simulink model "cllc_plant"  (R2020b)
settings: Solver=FixedStepDiscrete  StartTime=0.0  StopTime=Inf  FixedStep=stepsize  RelTol=1e-3  EnableMultiTasking=on
values from neighbouring files (symbols this model uses):
  Lm1 = Ln*LrP1    (= 0.00016)    [CLLC_Plant_Parameters.m]
  n = 20.0/9.0    (= 2.22222222222)    [CLLC_Plant_Parameters.m]
  stepsize = 2.0E-7    [cllc_data_lib.sldd]
  var_dir_v2g = 0.0    [cllc_data_lib.sldd]
  var_ref_iout = 18.5    [cllc_data_lib.sldd]
  var_ref_vout = 250.0    [cllc_data_lib.sldd]
libraries: fl_lib x219, ee_lib x151, nesl_utility x117, powerlib_meascontrol x15, eeStairGenerator x1
(part 7 of 8)

== system cllc_plant/cllc2/QDsec ==
  VGS : Inport
  Controlled Voltage Source : fl_lib/Electrical/Electrical Sources/Controlled Voltage Source
  Diode3 : ee_lib/Semiconductors & Converters/Diode  Commented=on  ModelType=ee.enum.diode.modelType.pwl  IfMat=[.07, .12, .19, 1.75, 4.24, 7.32, 11.2; .16, .3, .72, 2.14, 4.02, 6.35, 9.12] A  TjVec=[25, 125] degC  VfVec=[.5, .7, .9, 1.3, 1.7, 2.1, 2.5] V  Vf=0.6 V  Ron=0.3 Ohm  Goff=1e-8 S  prmExp=ee.enum.diode.expParam.useTwo  I12=[.0137, .545] A  V12=[.6, .7] V  IS=1e-12 A  ec=1  I1=0.0137 A  V1=0.6 V  RS=0 Ohm  Tmeas=25 degC  N_series=1  N_parallel=1  Rz=0.3 Ohm  BV=inf V  C_param=ee.enum.diode.capParam.fixed  CJ=5 pF  CJ0=5 pF  VJ=1 V  Mgrad=0.5  Vvec=[.1, 10, 100] V  Cvec=[3.5, 1, .4] pF  FC=0.5  Q_param=ee.enum.diode.recoveryParam.off  iRM=-7.15 A  iF=4 A  didt=-750 A/us  trr_factor=3  trr=115 ns  Qrr=1500 s*uA  TT=50 ns  tau=100 ns  T_param=ee.enum.diode.temperatureParam.off  IS_T2=1.25e-7 A  I1_T2=0.245 A  V1_T2=0.5 V  Tmeas2=125 degC  EG_param=ee.enum.diode.egapParam.material_si  EG=1.11 eV  XTI_param=ee.enum.diode.xtiParam.pn  XTI=3  dBVdT=0 V/K  Tdevice=25 degC  i_specify=off  i_priority=None  i=0 A  i_nominal_specify=off  i_nominal_unit=A  i_nominal_value=1  v_specify=off  v_priority=None  v=0 V  v_nominal_specify=off  v_nominal_unit=V  v_nominal_value=1  i_capacitor_specify=off  i_capacitor_priority=None  i_capacitor=0 A  i_capacitor_nominal_specify=off  i_capacitor_nominal_unit=A  i_capacitor_nominal_value=1  v_capacitor_specify=off  v_capacitor_priority=None  v_capacitor=0 V  v_capacitor_nominal_specify=off  v_capacitor_nominal_unit=V  v_capacitor_nominal_value=1  power_dissipated_specify=off  power_dissipated_priority=None  power_dissipated=0 W  power_dissipated_nominal_specify=off  power_dissipated_nominal_unit=W  power_dissipated_nominal_value=1  thermal_network_parameterization=ee.enum.thermalNetworkTopology.cauer  Rth=[0, 10] K/W  Rth_Foster=[4, 6] K/W  thermal_mass_parameterization=ee.enum.thermalNetwork.timeconstant  thermal_mass=[0, 1] J/K  thermal_mass_Foster=[1.5, 3] J/K  thermal_time_constant=[0, 10] s  thermal_time_constant_Foster=[6, 18] s  thermal_mass_initial_temperatures=[25, 25] degC
  F4-23MR12W1M1_B9 : ee_lib/Semiconductors & Converters/N-Channel MOSFET  paramTerminal=ee.enum.mosfet.numberOfTerminals.three  parameterization=1  prmDatasheet=2  prmEquCoeff=1  Beta=5.0 A/V^2  Rds=0.0225 Ohm  Id=50 A  Vgs=15 V  Vth=4.5 V  Vth0=1.7 V  lam=0 1/V  gamma_vth=0.5 V^0.50000  phib=0.5 V  Vth1=1.9071 V  Vbs1=-1 V  Vth2=2.066 V  Vbs2=-2 V  Tmeas=25 degC  RS=0.0001 Ohm  RD=0.0001 Ohm  RB=0.001 Ohm  C_param=1  C_GS=270 pF  C_GD=80 pF  C_DS=0 pF  C_iss=3.68 nF  C_rss=0.028 nF  C_oss=0.22 nF  charge_linearity_param=2  C_OX=200 pF  V_C_OX=-0.5 V  C_iss_vec=[2200,2000,1950,1900,1900,1900,1900,1900,1900,1900,1900,1900,1900,1900,1900,1900,1900,1900,1900,1900,1900] pF  C_rss_vec=[400,200,65,50,43,38,35,33,31,29,28,27,21,18,16,15,14,14,14,14,14] pF  C_oss_vec=[1900,1200,700,550,450,400,350,340,310,290,280,260,200,160,140,120,120,115,110,110,110] pF  C_GS_vec=[270, 300, 290, 280, 295, 255] pF  C_GD_vec=[450, 400, 300, 190, 95, 55] pF  C_DS_vec=[450, 410, 390, 230, 175, 115] pF  C_Vds_vec=[1,5,10,20,30,40,50,60,70,80,90,100,200,300,400,500,600,700,800,900,1000] V  V_GS_for_cap_data=0 V  charge_linearity_param_vgb=ee.enum.mosfet.cgbLinearity.instantly  IsDiode=0 A  Vbi=4.6 V  n=1  Cj0Diode=0 nF  TT=50e-9 s  dVth_dT=-6 mV/K  dVth0_dT=-6 mV/K  Rds_T2=0.033 Ohm  Tmeas2=150 degC  BEXDatasheet=-1.5  BEXEquCoeff=-1.5  etaisDatasheet=3  etaisEquCoeff=3  TdeviceDatasheet=25 degC  TdeviceEquCoeff=25 degC  thermal_network_parameterization=ee.enum.thermalNetworkTopology.cauer  Rth=[0.51, 10] K/W  Rth_Foster=[4, 6] K/W  thermal_mass_parameterization=ee.enum.thermalNetwork.timeconstant  thermal_mass=[0, 1] J/K  thermal_mass_Foster=[1.5, 3] J/K  thermal_time_constant=[0, 10] s  thermal_time_constant_Foster=[6, 18] s  thermal_mass_initial_temperatures=[25, 25] degC  betaref=18 A/V^2  Vfbref=-1.1 V  gamma=3.5 V^0.50000  phib2ref=1 V  thesatref=0.4 1/V  alpha=0  Vp=5e-2 V  thesrref=0 1/V  m=8  Tref=25 degC  Cox=1500 pF  Cgso=100 pF  Cgdo=14 pF  Rsref=2e-3 Ohm  Rdref=0.17 Ohm  Rgref=8.4 Ohm  Rbref=2e-3 Ohm  Isref=5.2e-13 A  Cj0=480 pF  Tprm=1  etabet=1.3  Stvfb=5e-4 V/K  Stphib=-8.5e-4 V/K  etasat=1.04  etasr=0.65  etar=0.95  etais=3  Tsim=25 degC  T0=[25, 25] degC
      settings: LogSimulationData=on
  ILm9 : fl_lib/Electrical/Electrical Sensors/Current Sensor
  PS-Simulink Converter22 : nesl_utility/PS-Simulink Converter  PhysicalDomain=network_engine_domain  SubClassName=ps_output  LeftPortType=input  RightPortType=output  PseudoPeriodic=off  Frequencies=[]  Unit=1  AffineConversion=off
  PS-Simulink Converter25 : nesl_utility/PS-Simulink Converter  PhysicalDomain=network_engine_domain  SubClassName=ps_output  LeftPortType=input  RightPortType=output  PseudoPeriodic=off  Frequencies=[]  Unit=1  AffineConversion=off
  Rg : ee_lib/Passive/Resistor  R=2 Ohm  R_tol=1  enable_R_tol=0  tol_distribution=1  nSigma=4  enable_operating_limits=0  operating_limit_action=2  max_working_voltage=100 V  power_rating=1 W  enable_faults=0  fault_action=1  R_faulted=inf Ohm  enable_temporal_fault=0  t_fault=1 s  enable_behavioral_fault=0  max_permissible_current=1 A  t_fail_on_current=1 s  noise_mode=0  sample_time=1e-3 s  repeatability=1  auto_seed=2919300768  user_seed=0  Tdevice=25 degC  alpha=3.93e-3 1/K  Tmeas=25 degC  thermal_mass=100 J/K  power_derating_T1=70 degC  power_derating_T2=155 degC  operating_temperature_range_vec=[-50, 150] degC  temperature_specify=off  temperature_priority=High  temperature=298.15 K  temperature_nominal_specify=off  temperature_nominal_unit=K  temperature_nominal_value=1
  Simulink-PS Converter2 : nesl_utility/Simulink-PS Converter  PhysicalDomain=network_engine_domain  SubClassName=ps_input  LeftPortType=input  RightPortType=output  PseudoPeriodic=off  Frequencies=[]  NoiseDistribution=none  NoiseParameters=[]  Unit=1  AffineConversion=off  FilteringAndDerivatives=provide  SimscapeFilterOrder=1  InputFilterTimeConstant=0.001  UdotUserProvided=0
  Voltage Sensor17 : fl_lib/Electrical/Electrical Sensors/Voltage Sensor
  + : PMIOPort  Side=Left
  - : PMIOPort  Port=2  Side=Left
  VDS : Outport  VectorParamsAs1DForOutWhenUnconnected=off
  IDS : Outport  Port=2  VectorParamsAs1DForOutWhenUnconnected=off
  wires:
  PS-Simulink Converter22/1 -> IDS/1
  PS-Simulink Converter25/1 -> VDS/1
  VGS/1 -> Simulink-PS Converter2/1
  connections:
  F4-23MR12W1M1_B9/LConn1 -- Rg/RConn1
  F4-23MR12W1M1_B9/RConn1 -- ILm9/RConn2 -- Voltage Sensor17/LConn1 -- Diode3/RConn1
  +/RConn1 -- ILm9/LConn1
  Controlled Voltage Source/RConn2 -- F4-23MR12W1M1_B9/RConn2 -- Voltage Sensor17/RConn2 -- Diode3/LConn1 -- -/RConn1
  PS-Simulink Converter22/LConn1 -- ILm9/RConn1
  PS-Simulink Converter25/LConn1 -- Voltage Sensor17/RConn1
  Rg/LConn1 -- Controlled Voltage Source/LConn1
  Controlled Voltage Source/RConn1 -- Simulink-PS Converter2/RConn1

== system cllc_plant/cllc2/tank_current_pri ==
  note: 1) Add Subsystem or Model blocks as valid variant choices.
      | 2) You cannot connect blocks at this level. At simulation, connectivity is automatically
      | determined, based on the active variant and port name matching.
  G2V : Subsystem  VariantControl=var_dir_v2g==0
  V2G : Subsystem  VariantControl=var_dir_v2g==1
  L : PMIOPort  Side=Left
  R : PMIOPort  Port=2  Side=Left
  to_scope : Outport

== system cllc_plant/cllc2/tank_current_sec ==
  note: 1) Add Subsystem or Model blocks as valid variant choices.
      | 2) You cannot connect blocks at this level. At simulation, connectivity is automatically
      | determined, based on the active variant and port name matching.
  G2V : Subsystem  VariantControl=var_dir_v2g==0
  V2G : Subsystem  VariantControl=var_dir_v2g==1
  L : PMIOPort  Side=Left
  R : PMIOPort  Port=2  Side=Left
  to_scope : Outport

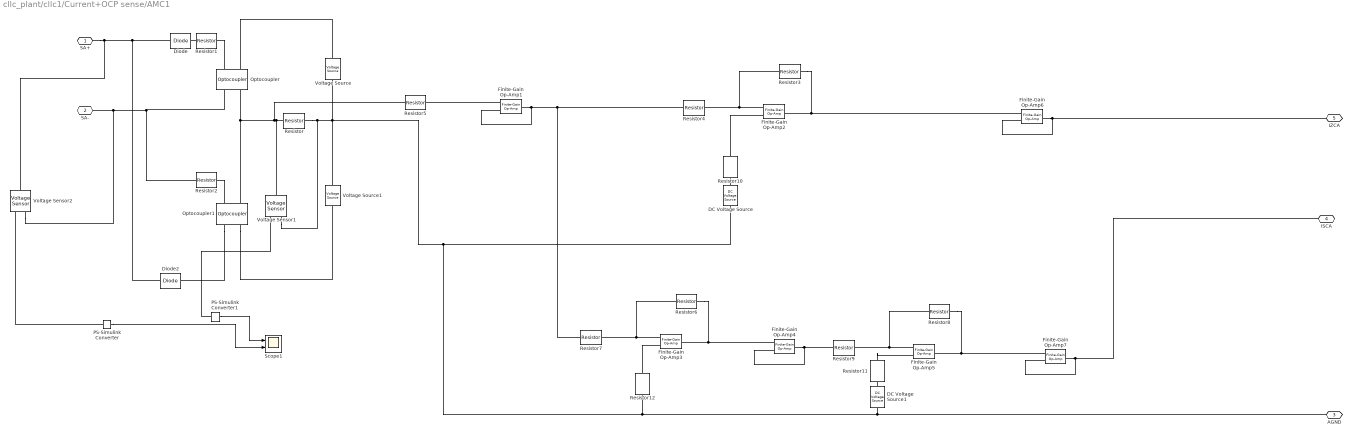
== system cllc_plant/cllc1/Current+OCP sense/AMC1 ==
  DC Voltage Source : fl_lib/Electrical/Electrical Sources/DC Voltage Source  v0=0.745 V
  DC Voltage Source1 : fl_lib/Electrical/Electrical Sources/DC Voltage Source  v0=0.745 V
  Diode : fl_lib/Electrical/Electrical Elements/Diode  Vf=0.000001 V  Ron=0.0000001 Ohm  Goff=1e-8 1/Ohm  i_specify=off  i_priority=None  i=0 A  i_nominal_specify=off  i_nominal_unit=A  i_nominal_value=1  v_specify=off  v_priority=None  v=0 V  v_nominal_specify=off  v_nominal_unit=V  v_nominal_value=1
  Diode2 : fl_lib/Electrical/Electrical Elements/Diode  Vf=0.000001 V  Ron=0.0000001 Ohm  Goff=1e-8 1/Ohm  i_specify=off  i_priority=None  i=0 A  i_nominal_specify=off  i_nominal_unit=A  i_nominal_value=1  v_specify=off  v_priority=None  v=0 V  v_nominal_specify=off  v_nominal_unit=V  v_nominal_value=1
  Finite-Gain Op-Amp1 : ee_lib/Integrated Circuits/Finite-Gain Op-Amp  A=1000  Rin=1e6 Ohm  Rout=100 Ohm  Vmin=-3.65 V  Vmax=3.65 V  noise_mode=0  v_noise=30e-9 V/Hz^0.50000  noise_prm=1  i_noise=0.5e-12 A/Hz^0.50000  ip_noise=0.5e-12 A/Hz^0.50000  in_noise=0.5e-12 A/Hz^0.50000  sample_time=1e-3 s  repeatability=1  auto_seed_v=3726858180  auto_seed_ip=508128604  auto_seed_in=167602409  user_seed_v=0  user_seed_ip=0  user_seed_in=0
      settings: SourceProductBaseCode=PS  InternalSimscapePortConfiguration="{\"Bottom\":[],\"Left\":[{\"id\":\"p\",\"label\":\"+\",\"type\":\"foundation.electrical.electrical\"},{\"id\":\"n\",\"label\":\"-\",\"type\":\"foundation.electrical.electrical\"}],\"Right\":[{\"id\":\"out\",\"label\":\"\",\"type\":\"foundation.electrical.electrical\"}],\"Top\":[]}"
  Finite-Gain Op-Amp2 : ee_lib/Integrated Circuits/Finite-Gain Op-Amp  A=1000  Rin=1e6 Ohm  Rout=100 Ohm  Vmin=0 V  Vmax=3.65 V  noise_mode=0  v_noise=30e-9 V/Hz^0.50000  noise_prm=1  i_noise=0.5e-12 A/Hz^0.50000  ip_noise=0.5e-12 A/Hz^0.50000  in_noise=0.5e-12 A/Hz^0.50000  sample_time=1e-3 s  repeatability=1  auto_seed_v=2569225923  auto_seed_ip=2595506743  auto_seed_in=2218060313  user_seed_v=0  user_seed_ip=0  user_seed_in=0
      settings: SourceProductBaseCode=PS  InternalSimscapePortConfiguration="{\"Bottom\":[],\"Left\":[{\"id\":\"p\",\"label\":\"+\",\"type\":\"foundation.electrical.electrical\"},{\"id\":\"n\",\"label\":\"-\",\"type\":\"foundation.electrical.electrical\"}],\"Right\":[{\"id\":\"out\",\"label\":\"\",\"type\":\"foundation.electrical.electrical\"}],\"Top\":[]}"
  Finite-Gain Op-Amp3 : ee_lib/Integrated Circuits/Finite-Gain Op-Amp  A=1000  Rin=1e6 Ohm  Rout=100 Ohm  Vmin=-3.65 V  Vmax=3.65 V  noise_mode=0  v_noise=30e-9 V/Hz^0.50000  noise_prm=1  i_noise=0.5e-12 A/Hz^0.50000  ip_noise=0.5e-12 A/Hz^0.50000  in_noise=0.5e-12 A/Hz^0.50000  sample_time=1e-3 s  repeatability=1  auto_seed_v=32244056  auto_seed_ip=2958946266  auto_seed_in=4063126573  user_seed_v=0  user_seed_ip=0  user_seed_in=0
      settings: SourceProductBaseCode=PS  InternalSimscapePortConfiguration="{\"Bottom\":[],\"Left\":[{\"id\":\"p\",\"label\":\"+\",\"type\":\"foundation.electrical.electrical\"},{\"id\":\"n\",\"label\":\"-\",\"type\":\"foundation.electrical.electrical\"}],\"Right\":[{\"id\":\"out\",\"label\":\"\",\"type\":\"foundation.electrical.electrical\"}],\"Top\":[]}"
  Finite-Gain Op-Amp4 : ee_lib/Integrated Circuits/Finite-Gain Op-Amp  A=1000  Rin=1e6 Ohm  Rout=100 Ohm  Vmin=-3.65 V  Vmax=3.65 V  noise_mode=0  v_noise=30e-9 V/Hz^0.50000  noise_prm=1  i_noise=0.5e-12 A/Hz^0.50000  ip_noise=0.5e-12 A/Hz^0.50000  in_noise=0.5e-12 A/Hz^0.50000  sample_time=1e-3 s  repeatability=1  auto_seed_v=3751810512  auto_seed_ip=486518659  auto_seed_in=1522863725  user_seed_v=0  user_seed_ip=0  user_seed_in=0
      settings: SourceProductBaseCode=PS  InternalSimscapePortConfiguration="{\"Bottom\":[],\"Left\":[{\"id\":\"p\",\"label\":\"+\",\"type\":\"foundation.electrical.electrical\"},{\"id\":\"n\",\"label\":\"-\",\"type\":\"foundation.electrical.electrical\"}],\"Right\":[{\"id\":\"out\",\"label\":\"\",\"type\":\"foundation.electrical.electrical\"}],\"Top\":[]}"
  Finite-Gain Op-Amp5 : ee_lib/Integrated Circuits/Finite-Gain Op-Amp  A=1000  Rin=1e6 Ohm  Rout=100 Ohm  Vmin=0 V  Vmax=3.65 V  noise_mode=0  v_noise=30e-9 V/Hz^0.50000  noise_prm=1  i_noise=0.5e-12 A/Hz^0.50000  ip_noise=0.5e-12 A/Hz^0.50000  in_noise=0.5e-12 A/Hz^0.50000  sample_time=1e-3 s  repeatability=1  auto_seed_v=1039110775  auto_seed_ip=2406613241  auto_seed_in=2631642888  user_seed_v=0  user_seed_ip=0  user_seed_in=0
      settings: SourceProductBaseCode=PS  InternalSimscapePortConfiguration="{\"Bottom\":[],\"Left\":[{\"id\":\"p\",\"label\":\"+\",\"type\":\"foundation.electrical.electrical\"},{\"id\":\"n\",\"label\":\"-\",\"type\":\"foundation.electrical.electrical\"}],\"Right\":[{\"id\":\"out\",\"label\":\"\",\"type\":\"foundation.electrical.electrical\"}],\"Top\":[]}"
  Finite-Gain Op-Amp6 : ee_lib/Integrated Circuits/Finite-Gain Op-Amp  A=1000  Rin=1e6 Ohm  Rout=100 Ohm  Vmin=-3.65 V  Vmax=3.65 V  noise_mode=0  v_noise=30e-9 V/Hz^0.50000  noise_prm=1  i_noise=0.5e-12 A/Hz^0.50000  ip_noise=0.5e-12 A/Hz^0.50000  in_noise=0.5e-12 A/Hz^0.50000  sample_time=1e-3 s  repeatability=1  auto_seed_v=1291965207  auto_seed_ip=3427992560  auto_seed_in=3417254766  user_seed_v=0  user_seed_ip=0  user_seed_in=0
      settings: SourceProductBaseCode=PS  InternalSimscapePortConfiguration="{\"Bottom\":[],\"Left\":[{\"id\":\"p\",\"label\":\"+\",\"type\":\"foundation.electrical.electrical\"},{\"id\":\"n\",\"label\":\"-\",\"type\":\"foundation.electrical.electrical\"}],\"Right\":[{\"id\":\"out\",\"label\":\"\",\"type\":\"foundation.electrical.electrical\"}],\"Top\":[]}"
  Finite-Gain Op-Amp7 : ee_lib/Integrated Circuits/Finite-Gain Op-Amp  A=1000  Rin=1e6 Ohm  Rout=100 Ohm  Vmin=-3.65 V  Vmax=3.65 V  noise_mode=0  v_noise=30e-9 V/Hz^0.50000  noise_prm=1  i_noise=0.5e-12 A/Hz^0.50000  ip_noise=0.5e-12 A/Hz^0.50000  in_noise=0.5e-12 A/Hz^0.50000  sample_time=1e-3 s  repeatability=1  auto_seed_v=3354765737  auto_seed_ip=1507956285  auto_seed_in=233205360  user_seed_v=0  user_seed_ip=0  user_seed_in=0
      settings: SourceProductBaseCode=PS  InternalSimscapePortConfiguration="{\"Bottom\":[],\"Left\":[{\"id\":\"p\",\"label\":\"+\",\"type\":\"foundation.electrical.electrical\"},{\"id\":\"n\",\"label\":\"-\",\"type\":\"foundation.electrical.electrical\"}],\"Right\":[{\"id\":\"out\",\"label\":\"\",\"type\":\"foundation.electrical.electrical\"}],\"Top\":[]}"
  Optocoupler : ee_lib/Semiconductors & Converters/Optocoupler  CTR=8.2  prmExp=1  I12=[.001, .002] A  V12=[0.000001, 0.000002] V  IS=1e-10 A  ec=2  RS=0.000001 Ohm  Tmeas=25 degC  C_param=1  CJ=0.000001 pF  CJ0=5 pF  VJ=1 V  Mgrad=0.5  Vvec=[.1, 10, 100] V  Cvec=[3.5, 1, .4] pF  FC=0.5  T_param=1  IS_T2=1.8e-8 A  I1_T2=0.029 A  V1_T2=1.05 V  Tmeas2=125 degC  EG_param=1  EG=1.11 eV  XTI_param=1  XTI=3  Tdevice=25 degC  i_capacitor_specify=off  i_capacitor_priority=High  i_capacitor=0 A  i_capacitor_nominal_specify=off  i_capacitor_nominal_unit=A  i_capacitor_nominal_value=1  v_capacitor_specify=off  v_capacitor_priority=None  v_capacitor=0 V  v_capacitor_nominal_specify=off  v_capacitor_nominal_unit=V  v_capacitor_nominal_value=1  thermal_network_parameterization=ee.enum.thermalNetworkTopology.cauer  Rth=[0, 10] K/W  Rth_Foster=[4, 6] K/W  thermal_mass_parameterization=ee.enum.thermalNetwork.timeconstant  thermal_mass=[0, 1] J/K  thermal_mass_Foster=[1.5, 3] J/K  thermal_time_constant=[0, 10] s  thermal_time_constant_Foster=[6, 18] s  thermal_mass_initial_temperatures=[25, 25] degC
      settings: SourceProductBaseCode=PS  InternalSimscapePortConfiguration="{\"Bottom\":[],\"Left\":[{\"id\":\"p\",\"label\":\"\",\"type\":\"foundation.electrical.electrical\"},{\"id\":\"C\",\"label\":\"\",\"type\":\"foundation.electrical.electrical\"}],\"Right\":[{\"id\":\"n\",\"label\":\"\",\"type\":\"foundation.electrical.electrical\"},{\"id\":\"E\",\"label\":\"\",\"type\":\"foundation.electrical.electrical\"}],\"Top\":[]}"
  Optocoupler1 : ee_lib/Semiconductors & Converters/Optocoupler  CTR=8.2  prmExp=1  I12=[.001, .002] A  V12=[0.000001, 0.000002] V  IS=1e-10 A  ec=2  RS=0.000001 Ohm  Tmeas=25 degC  C_param=1  CJ=0.000001 pF  CJ0=5 pF  VJ=1 V  Mgrad=0.5  Vvec=[.1, 10, 100] V  Cvec=[3.5, 1, .4] pF  FC=0.5  T_param=1  IS_T2=1.8e-8 A  I1_T2=0.029 A  V1_T2=1.05 V  Tmeas2=125 degC  EG_param=1  EG=1.11 eV  XTI_param=1  XTI=3  Tdevice=25 degC  i_capacitor_specify=off  i_capacitor_priority=High  i_capacitor=0 A  i_capacitor_nominal_specify=off  i_capacitor_nominal_unit=A  i_capacitor_nominal_value=1  v_capacitor_specify=off  v_capacitor_priority=None  v_capacitor=0 V  v_capacitor_nominal_specify=off  v_capacitor_nominal_unit=V  v_capacitor_nominal_value=1  thermal_network_parameterization=ee.enum.thermalNetworkTopology.cauer  Rth=[0, 10] K/W  Rth_Foster=[4, 6] K/W  thermal_mass_parameterization=ee.enum.thermalNetwork.timeconstant  thermal_mass=[0, 1] J/K  thermal_mass_Foster=[1.5, 3] J/K  thermal_time_constant=[0, 10] s  thermal_time_constant_Foster=[6, 18] s  thermal_mass_initial_temperatures=[25, 25] degC
      settings: SourceProductBaseCode=PS  InternalSimscapePortConfiguration="{\"Bottom\":[],\"Left\":[{\"id\":\"p\",\"label\":\"\",\"type\":\"foundation.electrical.electrical\"},{\"id\":\"C\",\"label\":\"\",\"type\":\"foundation.electrical.electrical\"}],\"Right\":[{\"id\":\"n\",\"label\":\"\",\"type\":\"foundation.electrical.electrical\"},{\"id\":\"E\",\"label\":\"\",\"type\":\"foundation.electrical.electrical\"}],\"Top\":[]}"
  PS-Simulink Converter : nesl_utility/PS-Simulink Converter  PhysicalDomain=network_engine_domain  SubClassName=ps_output  LeftPortType=input  RightPortType=output  PseudoPeriodic=off  Frequencies=[]  Unit=1  AffineConversion=off
  PS-Simulink Converter1 : nesl_utility/PS-Simulink Converter  PhysicalDomain=network_engine_domain  SubClassName=ps_output  LeftPortType=input  RightPortType=output  PseudoPeriodic=off  Frequencies=[]  Unit=1  AffineConversion=off
  Resistor : fl_lib/Electrical/Electrical Elements/Resistor  R=50 Ohm  i_specify=off  i_priority=None  i=0 A  i_nominal_specify=off  i_nominal_unit=A  i_nominal_value=1  v_specify=off  v_priority=None  v=0 V  v_nominal_specify=off  v_nominal_unit=V  v_nominal_value=1
  Resistor1 : fl_lib/Electrical/Electrical Elements/Resistor  R=100 Ohm  i_specify=off  i_priority=None  i=0 A  i_nominal_specify=off  i_nominal_unit=A  i_nominal_value=1  v_specify=off  v_priority=None  v=0 V  v_nominal_specify=off  v_nominal_unit=V  v_nominal_value=1
  Resistor{3..12} (10 alike) : fl_lib/Electrical/Electrical Elements/Resistor  R=1000 Ohm  i_specify=off  i_priority=None  i=0 A  i_nominal_specify=off  i_nominal_unit=A  i_nominal_value=1  v_specify=off  v_priority=None  v=0 V  v_nominal_specify=off  v_nominal_unit=V  v_nominal_value=1
  Resistor2 : fl_lib/Electrical/Electrical Elements/Resistor  R=100 Ohm  i_specify=off  i_priority=None  i=0 A  i_nominal_specify=off  i_nominal_unit=A  i_nominal_value=1  v_specify=off  v_priority=None  v=0 V  v_nominal_specify=off  v_nominal_unit=V  v_nominal_value=1
  Scope1 : Scope  NumInputPorts=2
  Voltage Sensor1 : fl_lib/Electrical/Electrical Sensors/Voltage Sensor
  Voltage Sensor2 : fl_lib/Electrical/Electrical Sensors/Voltage Sensor
  Voltage Source : ee_lib/Sources/Voltage Source  dc_voltage=3.6 V  ac_voltage=0 V  ac_shift=0 rad  ac_frequency=60 Hz  noise_mode=0  PSD=0 V^2/Hz  repeatability=1  auto_seed=3043863152  user_seed=0  sample_time=1e-3 s  i_specify=off  i_priority=None  i=0 A  i_nominal_specify=off  i_nominal_unit=A  i_nominal_value=1  v_specify=off  v_priority=None  v=0 V  v_nominal_specify=off  v_nominal_unit=V  v_nominal_value=1
  Voltage Source1 : ee_lib/Sources/Voltage Source  dc_voltage=3.6 V  ac_voltage=0 V  ac_shift=0 rad  ac_frequency=60 Hz  noise_mode=0  PSD=0 V^2/Hz  repeatability=1  auto_seed=4264595182  user_seed=0  sample_time=1e-3 s  i_specify=off  i_priority=None  i=0 A  i_nominal_specify=off  i_nominal_unit=A  i_nominal_value=1  v_specify=off  v_priority=None  v=0 V  v_nominal_specify=off  v_nominal_unit=V  v_nominal_value=1
  SA+ : PMIOPort  Side=Left
  SA- : PMIOPort  Port=2  Side=Left
  AGND : PMIOPort  Port=3  Side=Left
  ISCA : PMIOPort  Port=4  Side=Right
  IZCA : PMIOPort  Port=5  Side=Right
  wires:
  PS-Simulink Converter1/1 -> Scope1/1
  PS-Simulink Converter/1 -> Scope1/2
  connections:
  Resistor7/RConn1 -- Resistor6/LConn1 -- Finite-Gain Op-Amp3/LConn2
  Resistor2/RConn1 -- Optocoupler1/LConn1
  Diode2/RConn1 -- Diode/LConn1 -- SA+/RConn1 -- Voltage Sensor2/LConn1
  Resistor6/RConn1 -- Finite-Gain Op-Amp4/LConn1 -- Finite-Gain Op-Amp3/RConn1
  Finite-Gain Op-Amp1/RConn1 -- Resistor4/LConn1 -- Resistor7/LConn1 -- Finite-Gain Op-Amp1/LConn2
  ISCA/RConn1 -- Finite-Gain Op-Amp7/RConn1 -- Finite-Gain Op-Amp7/LConn2
  SA-/RConn1 -- Resistor2/LConn1 -- Optocoupler/RConn1 -- Voltage Sensor2/RConn2
  Resistor1/LConn1 -- Diode/RConn1
  Finite-Gain Op-Amp2/LConn2 -- Resistor4/RConn1 -- Resistor3/LConn1
  Optocoupler1/RConn1 -- Diode2/LConn1
  Resistor1/RConn1 -- Optocoupler/LConn1
  IZCA/RConn1 -- Finite-Gain Op-Amp6/LConn2 -- Finite-Gain Op-Amp6/RConn1
  Optocoupler1/RConn2 -- Voltage Source1/RConn1
  Resistor10/LConn1 -- Finite-Gain Op-Amp2/LConn1
  Finite-Gain Op-Amp4/LConn2 -- Resistor9/LConn1 -- Finite-Gain Op-Amp4/RConn1
  Optocoupler1/LConn2 -- Optocoupler/RConn2 -- Resistor5/LConn1 -- Resistor/LConn1 -- Voltage Sensor1/LConn1
  Voltage Source/LConn1 -- Optocoupler/LConn2
  Resistor3/RConn1 -- Finite-Gain Op-Amp6/LConn1 -- Finite-Gain Op-Amp2/RConn1
  Resistor9/RConn1 -- Resistor8/LConn1 -- Finite-Gain Op-Amp5/LConn2
  Finite-Gain Op-Amp1/LConn1 -- Resistor5/RConn1
  Resistor8/RConn1 -- Finite-Gain Op-Amp7/LConn1 -- Finite-Gain Op-Amp5/RConn1
  Resistor12/LConn1 -- Finite-Gain Op-Amp3/LConn1
  PS-Simulink Converter/LConn1 -- Voltage Sensor2/RConn1
  PS-Simulink Converter1/LConn1 -- Voltage Sensor1/RConn1
  DC Voltage Source/LConn1 -- Resistor10/RConn1
  Resistor11/RConn1 -- DC Voltage Source1/LConn1
  Resistor11/LConn1 -- Finite-Gain Op-Amp5/LConn1
  DC Voltage Source/RConn1 -- AGND/RConn1 -- DC Voltage Source1/RConn1 -- Resistor12/RConn1 -- Voltage Source/RConn1 -- Voltage Source1/LConn1 -- Resistor/RConn1 -- Voltage Sensor1/RConn2

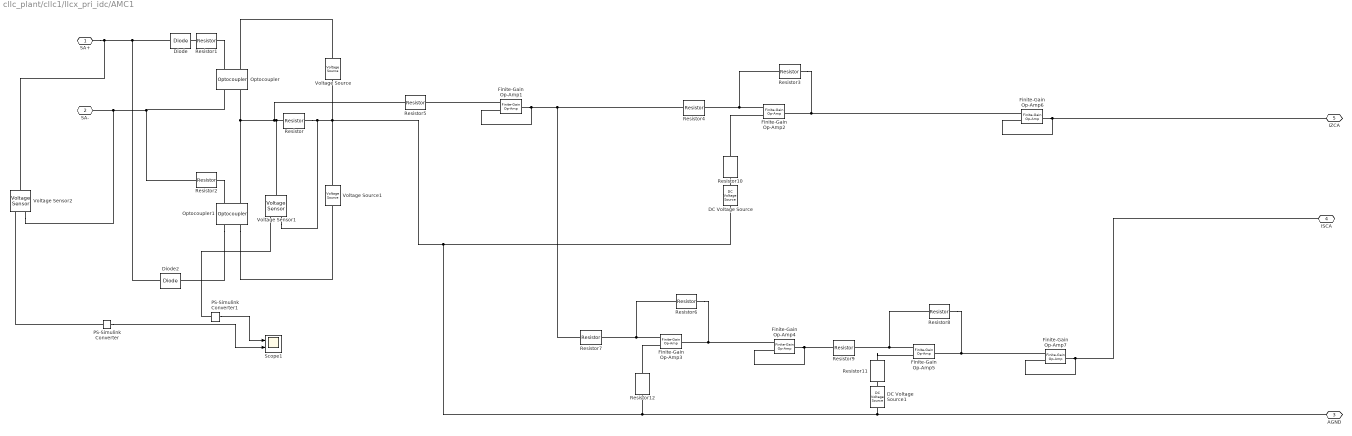
== system cllc_plant/cllc1/llcx_pri_idc/AMC1 ==
  DC Voltage Source : fl_lib/Electrical/Electrical Sources/DC Voltage Source  v0=0.745 V
  DC Voltage Source1 : fl_lib/Electrical/Electrical Sources/DC Voltage Source  v0=0.745 V
  Diode : fl_lib/Electrical/Electrical Elements/Diode  Vf=0.000001 V  Ron=0.0000001 Ohm  Goff=1e-8 1/Ohm  i_specify=off  i_priority=None  i=0 A  i_nominal_specify=off  i_nominal_unit=A  i_nominal_value=1  v_specify=off  v_priority=None  v=0 V  v_nominal_specify=off  v_nominal_unit=V  v_nominal_value=1
  Diode2 : fl_lib/Electrical/Electrical Elements/Diode  Vf=0.000001 V  Ron=0.0000001 Ohm  Goff=1e-8 1/Ohm  i_specify=off  i_priority=None  i=0 A  i_nominal_specify=off  i_nominal_unit=A  i_nominal_value=1  v_specify=off  v_priority=None  v=0 V  v_nominal_specify=off  v_nominal_unit=V  v_nominal_value=1
  Finite-Gain Op-Amp1 : ee_lib/Integrated Circuits/Finite-Gain Op-Amp  A=1000  Rin=1e6 Ohm  Rout=100 Ohm  Vmin=-3.65 V  Vmax=3.65 V  noise_mode=0  v_noise=30e-9 V/Hz^0.50000  noise_prm=1  i_noise=0.5e-12 A/Hz^0.50000  ip_noise=0.5e-12 A/Hz^0.50000  in_noise=0.5e-12 A/Hz^0.50000  sample_time=1e-3 s  repeatability=1  auto_seed_v=1126221968  auto_seed_ip=2489334968  auto_seed_in=3772388742  user_seed_v=0  user_seed_ip=0  user_seed_in=0
      settings: SourceProductBaseCode=PS  InternalSimscapePortConfiguration="{\"Bottom\":[],\"Left\":[{\"id\":\"p\",\"label\":\"+\",\"type\":\"foundation.electrical.electrical\"},{\"id\":\"n\",\"label\":\"-\",\"type\":\"foundation.electrical.electrical\"}],\"Right\":[{\"id\":\"out\",\"label\":\"\",\"type\":\"foundation.electrical.electrical\"}],\"Top\":[]}"
  Finite-Gain Op-Amp2 : ee_lib/Integrated Circuits/Finite-Gain Op-Amp  A=1000  Rin=1e6 Ohm  Rout=100 Ohm  Vmin=0 V  Vmax=3.65 V  noise_mode=0  v_noise=30e-9 V/Hz^0.50000  noise_prm=1  i_noise=0.5e-12 A/Hz^0.50000  ip_noise=0.5e-12 A/Hz^0.50000  in_noise=0.5e-12 A/Hz^0.50000  sample_time=1e-3 s  repeatability=1  auto_seed_v=261779212  auto_seed_ip=1893550016  auto_seed_in=361885361  user_seed_v=0  user_seed_ip=0  user_seed_in=0
      settings: SourceProductBaseCode=PS  InternalSimscapePortConfiguration="{\"Bottom\":[],\"Left\":[{\"id\":\"p\",\"label\":\"+\",\"type\":\"foundation.electrical.electrical\"},{\"id\":\"n\",\"label\":\"-\",\"type\":\"foundation.electrical.electrical\"}],\"Right\":[{\"id\":\"out\",\"label\":\"\",\"type\":\"foundation.electrical.electrical\"}],\"Top\":[]}"
  Finite-Gain Op-Amp3 : ee_lib/Integrated Circuits/Finite-Gain Op-Amp  A=1000  Rin=1e6 Ohm  Rout=100 Ohm  Vmin=-3.65 V  Vmax=3.65 V  noise_mode=0  v_noise=30e-9 V/Hz^0.50000  noise_prm=1  i_noise=0.5e-12 A/Hz^0.50000  ip_noise=0.5e-12 A/Hz^0.50000  in_noise=0.5e-12 A/Hz^0.50000  sample_time=1e-3 s  repeatability=1  auto_seed_v=2419087138  auto_seed_ip=2316321305  auto_seed_in=3298783563  user_seed_v=0  user_seed_ip=0  user_seed_in=0
      settings: SourceProductBaseCode=PS  InternalSimscapePortConfiguration="{\"Bottom\":[],\"Left\":[{\"id\":\"p\",\"label\":\"+\",\"type\":\"foundation.electrical.electrical\"},{\"id\":\"n\",\"label\":\"-\",\"type\":\"foundation.electrical.electrical\"}],\"Right\":[{\"id\":\"out\",\"label\":\"\",\"type\":\"foundation.electrical.electrical\"}],\"Top\":[]}"
  Finite-Gain Op-Amp4 : ee_lib/Integrated Circuits/Finite-Gain Op-Amp  A=1000  Rin=1e6 Ohm  Rout=100 Ohm  Vmin=-3.65 V  Vmax=3.65 V  noise_mode=0  v_noise=30e-9 V/Hz^0.50000  noise_prm=1  i_noise=0.5e-12 A/Hz^0.50000  ip_noise=0.5e-12 A/Hz^0.50000  in_noise=0.5e-12 A/Hz^0.50000  sample_time=1e-3 s  repeatability=1  auto_seed_v=1001115096  auto_seed_ip=2522699475  auto_seed_in=1971277748  user_seed_v=0  user_seed_ip=0  user_seed_in=0
      settings: SourceProductBaseCode=PS  InternalSimscapePortConfiguration="{\"Bottom\":[],\"Left\":[{\"id\":\"p\",\"label\":\"+\",\"type\":\"foundation.electrical.electrical\"},{\"id\":\"n\",\"label\":\"-\",\"type\":\"foundation.electrical.electrical\"}],\"Right\":[{\"id\":\"out\",\"label\":\"\",\"type\":\"foundation.electrical.electrical\"}],\"Top\":[]}"
  Finite-Gain Op-Amp5 : ee_lib/Integrated Circuits/Finite-Gain Op-Amp  A=1000  Rin=1e6 Ohm  Rout=100 Ohm  Vmin=0 V  Vmax=3.65 V  noise_mode=0  v_noise=30e-9 V/Hz^0.50000  noise_prm=1  i_noise=0.5e-12 A/Hz^0.50000  ip_noise=0.5e-12 A/Hz^0.50000  in_noise=0.5e-12 A/Hz^0.50000  sample_time=1e-3 s  repeatability=1  auto_seed_v=3697887478  auto_seed_ip=2838269414  auto_seed_in=1519899445  user_seed_v=0  user_seed_ip=0  user_seed_in=0
      settings: SourceProductBaseCode=PS  InternalSimscapePortConfiguration="{\"Bottom\":[],\"Left\":[{\"id\":\"p\",\"label\":\"+\",\"type\":\"foundation.electrical.electrical\"},{\"id\":\"n\",\"label\":\"-\",\"type\":\"foundation.electrical.electrical\"}],\"Right\":[{\"id\":\"out\",\"label\":\"\",\"type\":\"foundation.electrical.electrical\"}],\"Top\":[]}"
  Finite-Gain Op-Amp6 : ee_lib/Integrated Circuits/Finite-Gain Op-Amp  A=1000  Rin=1e6 Ohm  Rout=100 Ohm  Vmin=-3.65 V  Vmax=3.65 V  noise_mode=0  v_noise=30e-9 V/Hz^0.50000  noise_prm=1  i_noise=0.5e-12 A/Hz^0.50000  ip_noise=0.5e-12 A/Hz^0.50000  in_noise=0.5e-12 A/Hz^0.50000  sample_time=1e-3 s  repeatability=1  auto_seed_v=1491153795  auto_seed_ip=1089710952  auto_seed_in=4091077232  user_seed_v=0  user_seed_ip=0  user_seed_in=0
      settings: SourceProductBaseCode=PS  InternalSimscapePortConfiguration="{\"Bottom\":[],\"Left\":[{\"id\":\"p\",\"label\":\"+\",\"type\":\"foundation.electrical.electrical\"},{\"id\":\"n\",\"label\":\"-\",\"type\":\"foundation.electrical.electrical\"}],\"Right\":[{\"id\":\"out\",\"label\":\"\",\"type\":\"foundation.electrical.electrical\"}],\"Top\":[]}"
  Finite-Gain Op-Amp7 : ee_lib/Integrated Circuits/Finite-Gain Op-Amp  A=1000  Rin=1e6 Ohm  Rout=100 Ohm  Vmin=-3.65 V  Vmax=3.65 V  noise_mode=0  v_noise=30e-9 V/Hz^0.50000  noise_prm=1  i_noise=0.5e-12 A/Hz^0.50000  ip_noise=0.5e-12 A/Hz^0.50000  in_noise=0.5e-12 A/Hz^0.50000  sample_time=1e-3 s  repeatability=1  auto_seed_v=1280763499  auto_seed_ip=680348924  auto_seed_in=1551759043  user_seed_v=0  user_seed_ip=0  user_seed_in=0
      settings: SourceProductBaseCode=PS  InternalSimscapePortConfiguration="{\"Bottom\":[],\"Left\":[{\"id\":\"p\",\"label\":\"+\",\"type\":\"foundation.electrical.electrical\"},{\"id\":\"n\",\"label\":\"-\",\"type\":\"foundation.electrical.electrical\"}],\"Right\":[{\"id\":\"out\",\"label\":\"\",\"type\":\"foundation.electrical.electrical\"}],\"Top\":[]}"
  Optocoupler : ee_lib/Semiconductors & Converters/Optocoupler  CTR=8.2  prmExp=1  I12=[.001, .002] A  V12=[0.000001, 0.000002] V  IS=1e-10 A  ec=2  RS=0.000001 Ohm  Tmeas=25 degC  C_param=1  CJ=0.000001 pF  CJ0=5 pF  VJ=1 V  Mgrad=0.5  Vvec=[.1, 10, 100] V  Cvec=[3.5, 1, .4] pF  FC=0.5  T_param=1  IS_T2=1.8e-8 A  I1_T2=0.029 A  V1_T2=1.05 V  Tmeas2=125 degC  EG_param=1  EG=1.11 eV  XTI_param=1  XTI=3  Tdevice=25 degC  i_capacitor_specify=off  i_capacitor_priority=High  i_capacitor=0 A  i_capacitor_nominal_specify=off  i_capacitor_nominal_unit=A  i_capacitor_nominal_value=1  v_capacitor_specify=off  v_capacitor_priority=None  v_capacitor=0 V  v_capacitor_nominal_specify=off  v_capacitor_nominal_unit=V  v_capacitor_nominal_value=1  thermal_network_parameterization=ee.enum.thermalNetworkTopology.cauer  Rth=[0, 10] K/W  Rth_Foster=[4, 6] K/W  thermal_mass_parameterization=ee.enum.thermalNetwork.timeconstant  thermal_mass=[0, 1] J/K  thermal_mass_Foster=[1.5, 3] J/K  thermal_time_constant=[0, 10] s  thermal_time_constant_Foster=[6, 18] s  thermal_mass_initial_temperatures=[25, 25] degC
      settings: SourceProductBaseCode=PS  InternalSimscapePortConfiguration="{\"Bottom\":[],\"Left\":[{\"id\":\"p\",\"label\":\"\",\"type\":\"foundation.electrical.electrical\"},{\"id\":\"C\",\"label\":\"\",\"type\":\"foundation.electrical.electrical\"}],\"Right\":[{\"id\":\"n\",\"label\":\"\",\"type\":\"foundation.electrical.electrical\"},{\"id\":\"E\",\"label\":\"\",\"type\":\"foundation.electrical.electrical\"}],\"Top\":[]}"
  Optocoupler1 : ee_lib/Semiconductors & Converters/Optocoupler  CTR=8.2  prmExp=1  I12=[.001, .002] A  V12=[0.000001, 0.000002] V  IS=1e-10 A  ec=2  RS=0.000001 Ohm  Tmeas=25 degC  C_param=1  CJ=0.000001 pF  CJ0=5 pF  VJ=1 V  Mgrad=0.5  Vvec=[.1, 10, 100] V  Cvec=[3.5, 1, .4] pF  FC=0.5  T_param=1  IS_T2=1.8e-8 A  I1_T2=0.029 A  V1_T2=1.05 V  Tmeas2=125 degC  EG_param=1  EG=1.11 eV  XTI_param=1  XTI=3  Tdevice=25 degC  i_capacitor_specify=off  i_capacitor_priority=High  i_capacitor=0 A  i_capacitor_nominal_specify=off  i_capacitor_nominal_unit=A  i_capacitor_nominal_value=1  v_capacitor_specify=off  v_capacitor_priority=None  v_capacitor=0 V  v_capacitor_nominal_specify=off  v_capacitor_nominal_unit=V  v_capacitor_nominal_value=1  thermal_network_parameterization=ee.enum.thermalNetworkTopology.cauer  Rth=[0, 10] K/W  Rth_Foster=[4, 6] K/W  thermal_mass_parameterization=ee.enum.thermalNetwork.timeconstant  thermal_mass=[0, 1] J/K  thermal_mass_Foster=[1.5, 3] J/K  thermal_time_constant=[0, 10] s  thermal_time_constant_Foster=[6, 18] s  thermal_mass_initial_temperatures=[25, 25] degC
      settings: SourceProductBaseCode=PS  InternalSimscapePortConfiguration="{\"Bottom\":[],\"Left\":[{\"id\":\"p\",\"label\":\"\",\"type\":\"foundation.electrical.electrical\"},{\"id\":\"C\",\"label\":\"\",\"type\":\"foundation.electrical.electrical\"}],\"Right\":[{\"id\":\"n\",\"label\":\"\",\"type\":\"foundation.electrical.electrical\"},{\"id\":\"E\",\"label\":\"\",\"type\":\"foundation.electrical.electrical\"}],\"Top\":[]}"
  PS-Simulink Converter : nesl_utility/PS-Simulink Converter  PhysicalDomain=network_engine_domain  SubClassName=ps_output  LeftPortType=input  RightPortType=output  PseudoPeriodic=off  Frequencies=[]  Unit=1  AffineConversion=off
  PS-Simulink Converter1 : nesl_utility/PS-Simulink Converter  PhysicalDomain=network_engine_domain  SubClassName=ps_output  LeftPortType=input  RightPortType=output  PseudoPeriodic=off  Frequencies=[]  Unit=1  AffineConversion=off
  Resistor : fl_lib/Electrical/Electrical Elements/Resistor  R=50 Ohm  i_specify=off  i_priority=None  i=0 A  i_nominal_specify=off  i_nominal_unit=A  i_nominal_value=1  v_specify=off  v_priority=None  v=0 V  v_nominal_specify=off  v_nominal_unit=V  v_nominal_value=1
  Resistor1 : fl_lib/Electrical/Electrical Elements/Resistor  R=100 Ohm  i_specify=off  i_priority=None  i=0 A  i_nominal_specify=off  i_nominal_unit=A  i_nominal_value=1  v_specify=off  v_priority=None  v=0 V  v_nominal_specify=off  v_nominal_unit=V  v_nominal_value=1
  Resistor{3..12} (10 alike) : fl_lib/Electrical/Electrical Elements/Resistor  R=1000 Ohm  i_specify=off  i_priority=None  i=0 A  i_nominal_specify=off  i_nominal_unit=A  i_nominal_value=1  v_specify=off  v_priority=None  v=0 V  v_nominal_specify=off  v_nominal_unit=V  v_nominal_value=1
  Resistor2 : fl_lib/Electrical/Electrical Elements/Resistor  R=100 Ohm  i_specify=off  i_priority=None  i=0 A  i_nominal_specify=off  i_nominal_unit=A  i_nominal_value=1  v_specify=off  v_priority=None  v=0 V  v_nominal_specify=off  v_nominal_unit=V  v_nominal_value=1
  Scope1 : Scope  NumInputPorts=2
  Voltage Sensor1 : fl_lib/Electrical/Electrical Sensors/Voltage Sensor
  Voltage Sensor2 : fl_lib/Electrical/Electrical Sensors/Voltage Sensor
  Voltage Source : ee_lib/Sources/Voltage Source  dc_voltage=3.6 V  ac_voltage=0 V  ac_shift=0 rad  ac_frequency=60 Hz  noise_mode=0  PSD=0 V^2/Hz  repeatability=1  auto_seed=3185272699  user_seed=0  sample_time=1e-3 s  i_specify=off  i_priority=None  i=0 A  i_nominal_specify=off  i_nominal_unit=A  i_nominal_value=1  v_specify=off  v_priority=None  v=0 V  v_nominal_specify=off  v_nominal_unit=V  v_nominal_value=1
  Voltage Source1 : ee_lib/Sources/Voltage Source  dc_voltage=3.6 V  ac_voltage=0 V  ac_shift=0 rad  ac_frequency=60 Hz  noise_mode=0  PSD=0 V^2/Hz  repeatability=1  auto_seed=3031817457  user_seed=0  sample_time=1e-3 s  i_specify=off  i_priority=None  i=0 A  i_nominal_specify=off  i_nominal_unit=A  i_nominal_value=1  v_specify=off  v_priority=None  v=0 V  v_nominal_specify=off  v_nominal_unit=V  v_nominal_value=1
  SA+ : PMIOPort  Side=Left
  SA- : PMIOPort  Port=2  Side=Left
  AGND : PMIOPort  Port=3  Side=Left
  ISCA : PMIOPort  Port=4  Side=Right
  IZCA : PMIOPort  Port=5  Side=Right
  wires:
  PS-Simulink Converter1/1 -> Scope1/1
  PS-Simulink Converter/1 -> Scope1/2
  connections:
  Resistor7/RConn1 -- Resistor6/LConn1 -- Finite-Gain Op-Amp3/LConn2
  Resistor2/RConn1 -- Optocoupler1/LConn1
  Diode2/RConn1 -- Diode/LConn1 -- SA+/RConn1 -- Voltage Sensor2/LConn1
  Resistor6/RConn1 -- Finite-Gain Op-Amp4/LConn1 -- Finite-Gain Op-Amp3/RConn1
  Finite-Gain Op-Amp1/RConn1 -- Resistor4/LConn1 -- Resistor7/LConn1 -- Finite-Gain Op-Amp1/LConn2
  ISCA/RConn1 -- Finite-Gain Op-Amp7/RConn1 -- Finite-Gain Op-Amp7/LConn2
  SA-/RConn1 -- Resistor2/LConn1 -- Optocoupler/RConn1 -- Voltage Sensor2/RConn2
  Resistor1/LConn1 -- Diode/RConn1
  Finite-Gain Op-Amp2/LConn2 -- Resistor4/RConn1 -- Resistor3/LConn1
  Optocoupler1/RConn1 -- Diode2/LConn1
  Resistor1/RConn1 -- Optocoupler/LConn1
  IZCA/RConn1 -- Finite-Gain Op-Amp6/LConn2 -- Finite-Gain Op-Amp6/RConn1
  Optocoupler1/RConn2 -- Voltage Source1/RConn1
  Resistor10/LConn1 -- Finite-Gain Op-Amp2/LConn1
  Finite-Gain Op-Amp4/LConn2 -- Resistor9/LConn1 -- Finite-Gain Op-Amp4/RConn1
  Optocoupler1/LConn2 -- Optocoupler/RConn2 -- Resistor5/LConn1 -- Resistor/LConn1 -- Voltage Sensor1/LConn1
  Voltage Source/LConn1 -- Optocoupler/LConn2
  Resistor3/RConn1 -- Finite-Gain Op-Amp6/LConn1 -- Finite-Gain Op-Amp2/RConn1
  Resistor9/RConn1 -- Resistor8/LConn1 -- Finite-Gain Op-Amp5/LConn2
  Finite-Gain Op-Amp1/LConn1 -- Resistor5/RConn1
  Resistor8/RConn1 -- Finite-Gain Op-Amp7/LConn1 -- Finite-Gain Op-Amp5/RConn1
  Resistor12/LConn1 -- Finite-Gain Op-Amp3/LConn1
  PS-Simulink Converter/LConn1 -- Voltage Sensor2/RConn1
  PS-Simulink Converter1/LConn1 -- Voltage Sensor1/RConn1
  DC Voltage Source/LConn1 -- Resistor10/RConn1
  Resistor11/RConn1 -- DC Voltage Source1/LConn1
  Resistor11/LConn1 -- Finite-Gain Op-Amp5/LConn1
  DC Voltage Source/RConn1 -- AGND/RConn1 -- DC Voltage Source1/RConn1 -- Resistor12/RConn1 -- Voltage Source/RConn1 -- Voltage Source1/LConn1 -- Resistor/RConn1 -- Voltage Sensor1/RConn2

== system cllc_plant/cllc1/tank_current_pri/G2V ==
  Current Sensor2 : fl_lib/Electrical/Electrical Sensors/Current Sensor
  PS-Simulink Converter8 : nesl_utility/PS-Simulink Converter  PhysicalDomain=network_engine_domain  SubClassName=ps_output  LeftPortType=input  RightPortType=output  PseudoPeriodic=off  Frequencies=[]  Unit=1  AffineConversion=off
  L : PMIOPort  Side=Left
  R : PMIOPort  Port=2  Side=Left
  to_scope : Outport
  wires:
  PS-Simulink Converter8/1 -> to_scope/1
  connections:
  L/RConn1 -- Current Sensor2/LConn1
  Current Sensor2/RConn2 -- R/RConn1
  Current Sensor2/RConn1 -- PS-Simulink Converter8/LConn1

== system cllc_plant/cllc1/tank_current_pri/V2G ==
  Current Sensor2 : fl_lib/Electrical/Electrical Sensors/Current Sensor
  PS-Simulink Converter8 : nesl_utility/PS-Simulink Converter  PhysicalDomain=network_engine_domain  SubClassName=ps_output  LeftPortType=input  RightPortType=output  PseudoPeriodic=off  Frequencies=[]  Unit=1  AffineConversion=off
  L : PMIOPort  Side=Left
  R : PMIOPort  Port=2  Side=Left
  to_scope : Outport
  wires:
  PS-Simulink Converter8/1 -> to_scope/1
  connections:
  Current Sensor2/RConn2 -- L/RConn1
  Current Sensor2/RConn1 -- PS-Simulink Converter8/LConn1
  Current Sensor2/LConn1 -- R/RConn1

== system cllc_plant/cllc1/tank_current_sec/G2V ==
  Current Sensor2 : fl_lib/Electrical/Electrical Sensors/Current Sensor
  PS-Simulink Converter8 : nesl_utility/PS-Simulink Converter  PhysicalDomain=network_engine_domain  SubClassName=ps_output  LeftPortType=input  RightPortType=output  PseudoPeriodic=off  Frequencies=[]  Unit=1  AffineConversion=off
  L : PMIOPort  Side=Left
  R : PMIOPort  Port=2  Side=Left
  to_scope : Outport
  wires:
  PS-Simulink Converter8/1 -> to_scope/1
  connections:
  Current Sensor2/RConn1 -- PS-Simulink Converter8/LConn1
  Current Sensor2/RConn2 -- R/RConn1
  L/RConn1 -- Current Sensor2/LConn1

== system cllc_plant/cllc1/tank_current_sec/V2G ==
  Current Sensor2 : fl_lib/Electrical/Electrical Sensors/Current Sensor
  PS-Simulink Converter8 : nesl_utility/PS-Simulink Converter  PhysicalDomain=network_engine_domain  SubClassName=ps_output  LeftPortType=input  RightPortType=output  PseudoPeriodic=off  Frequencies=[]  Unit=1  AffineConversion=off
  L : PMIOPort  Side=Left
  R : PMIOPort  Port=2  Side=Left
  to_scope : Outport
  wires:
  PS-Simulink Converter8/1 -> to_scope/1
  connections:
  Current Sensor2/LConn1 -- R/RConn1
  Current Sensor2/RConn1 -- PS-Simulink Converter8/LConn1
  Current Sensor2/RConn2 -- L/RConn1
